simulink library "monroe_library"  (R2012b)
settings: Solver=ode45  StartTime=0.0  StopTime=10.0  RelTol=1e-3
values from neighbouring files (symbols this model uses):
  input_bit_width = ', num2str(input_bit_width))    [fft_direct_draw.m]
undefined symbols (not defined in the file or in its folder): gcbh, xlBlockLoadCallback
libraries: xbsIndex_r4 x1880, monroe_library x159, casper_library x13, xps_library x1
(part 42 of 43)

== system monroe_library/unscr_tail/mirror_spectrum/Subsystem3 ==
  In1 : Inport
  In3 : Inport  Port=2
  In4 : Inport  Port=3
  Delay11 : S-Function  LoadFcn=xlBlockLoadCallback(gcbh);  FunctionName=sysgen  Parameters=ptable_  EnableBusSupport=off  mask(Xilinx Delay Block){infoedit=Hardware notes: A delay line is a chain, each link of which is an SRL16 followed by a flip-flop., en_sgadvanced=, en=off, latency=1, dbl_ovrd_sgadvanced=, dbl_ovrd=off, reg_retiming_sgadvanced=, reg_retiming=off, xl_use_area_sgadvanced=, xl_use_area=off, xl_area=[0,0,0,0,0,0,0], has_advanced_control=0, sggui_pos=-1,-1,-1,-1, block_type=delay, block_version=, sg_icon_stat=25,28,1,1,white,blue,0,07b98262,right,,[ ],[ ], sg_mask_display=|, sg_list_contents=, sg_blockgui_xml=}
      mask sg_mask_display=|
      | fprintf('','COMMENT: begin icon graphics');
      | patch([0 25 25 0 0 ],[0 0 28 28 0 ],[0.77 0.82 0.91 ]);
      | plot([0 25 25 0 0 ],[0 0 28 28 0 ]);
      | patch([5.325 9.66 12.66 15.66 18.66 12.66 8.325 5.325 ],[17.33 17.33 20.33 17.33 20.33 20.33 20.33 17.33 ],[1 1 1 ]);
      | patch([8.325 12.66 9.66 5.325 8.325 ],[14.33 14.33 17.33 17.33 14.33 ],[0.931 0.946 0.973 ]);
      | patch([5.325 9.66 12.66 8.325 5.325 ],[11.33 11.33 14.33 14.33 11.33 ],[1 1 1 ]);
      | patch([8.325 18.66 15.66 12.66 9.66 5.325 8.325 ],[8.33 8.33 11.33 8.33 11.33 11.33 8.33 ],[0.931 0.946 0.973 ]);
      | fprintf('','COMMENT: end icon graphics');
      | fprintf('','COMMENT: begin icon text');
      |
      |
      | color('black');disp('z^{-1}','texmode','on');
      | fprintf('','COMMENT: end icon text');
      mask prompts: infoedit ""; en_sgadvanced ""; en "Provide enable port"; dbl_ovrd_sgadvanced ""; dbl_ovrd "Override with doubles"; reg_retiming_sgadvanced ""; reg_retiming "Implement using behavioral HDL."; xl_use_area_sgadvanced ""; xl_use_area "Define FPGA area for resource estimation"; xl_area "FPGA area [slices, FFs, BRAMs, LUTs, IOBs, emb. mults, TBUFs]"; has_advanced_control ""; sggui_pos ""; block_type ""; block_version ""; sg_icon_stat ""; sg_mask_display ""; sg_list_contents ""; sg_blockgui_xml ""
      mask help: Hardware notes: A delay line is a chain, each link of which is an SRL16 followed by a flip-flop.
      mask init: same as monroe_library/counter_limited_fast/Delay1
      settings: CopyFcn=xlBlockMoveCallback(gcbh);  DeleteFcn=xlDestroyGui(gcbh);  ModelCloseFcn=xlDestroyGui(gcbh);  PreSaveFcn=xlBlockPreSaveCallback(gcbh);  PostSaveFcn=xlBlockPostSaveCallback(gcbh);  DestroyFcn=xlDestroyGui(gcbh);  OpenFcn=xlOpenGui(gcbh, 'delay_gui.xml', @xlmagicenablement, -1)  CloseFcn=xlDestroyGui(gcbh);  MoveFcn=xlBlockMoveCallback(gcbh);
      mask Help: eval('');xlDoc('-book','sysgen','-topic','Delay');
      mask Display:
      | fprintf('','COMMENT: begin icon graphics');
      | patch([0 25 25 0 0 ],[0 0 28 28 0 ],[0.77 0.82 0.91 ]);
      | plot([0 25 25 0 0 ],[0 0 28 28 0 ]);
      | patch([5.325 9.66 12.66 15.66 18.66 12.66 8.325 5.325 ],[17.33 17.33 20.33 17.33 20.33 20.33 20.33 17.33 ],[1 1 1 ]);
      | patch([8.325 12.66 9.66 5.325 8.325 ],[14.33 14.33 17.33 17.33 14.33 ],[0.931 0.946 0.973 ]);
      | patch([5.325 9.66 12.66 8.325 5.325 ],[11.33 11.33 14.33 14.33 11.33 ],[1 1 1 ]);
      | patch([8.325 18.66 15.66 12.66 9.66 5.325 8.325 ],[8.33 8.33 11.33 8.33 11.33 11.33 8.33 ],[0.931 0.946 0.973 ]);
      | fprintf('','COMMENT: end icon graphics');
      | fprintf('','COMMENT: begin icon text');
      | 
      | 
      | color('black');disp('z^{-1}','texmode','on');
      | fprintf('','COMMENT: end icon text');
  Delay7 : xbsIndex_r4/Delay  en=off  latency=1  dbl_ovrd=off  reg_retiming=off  block_type=delay
  Mux4 : S-Function  LoadFcn=xlBlockLoadCallback(gcbh);  FunctionName=sysgen  Parameters=ptable_  EnableBusSupport=off  mask(Xilinx Bus Multiplexer Block){inputs_sgadvanced=, inputs=2, en_sgadvanced=, en=off, latency=0, precision_sgadvanced=, precision=Full, arith_type_sgadvanced=, arith_type=Signed  (2's comp), n_bits=8, bin_pt=2, quantization_sgadvanced=, quantization=Truncate, overflow_sgadvanced=, overflow=Wrap, dbl_ovrd_sgadvanced=, dbl_ovrd=off, xl_use_area_sgadvanced=, xl_use_area=off, xl_area=[0,0,0,0,0,0,0], infoedit=, has_advanced_control=0, sggui_pos=-1,-1,-1,-1, block_type=mux, block_version=, sg_icon_stat=45,104,3,1,white,blue,3,eb98d690,right,,[ ],[ ], sg_mask_display=|, sg_list_contents=, sg_blockgui_xml=}
      mask sg_mask_display=|
      | fprintf('','COMMENT: begin icon graphics');
      | patch([0 45 45 0 0 ],[0 14.8571 89.1429 104 0 ],[0.77 0.82 0.91 ]);
      | plot([0 45 45 0 0 ],[0 14.8571 89.1429 104 0 ]);
      | patch([8.65 17.32 23.32 29.32 35.32 23.32 14.65 8.65 ],[58.66 58.66 64.66 58.66 64.66 64.66 64.66 58.66 ],[1 1 1 ]);
      | patch([14.65 23.32 17.32 8.65 14.65 ],[52.66 52.66 58.66 58.66 52.66 ],[0.931 0.946 0.973 ]);
      | patch([8.65 17.32 23.32 14.65 8.65 ],[46.66 46.66 52.66 52.66 46.66 ],[1 1 1 ]);
      | patch([14.65 35.32 29.32 23.32 17.32 8.65 14.65 ],[40.66 40.66 46.66 40.66 46.66 46.66 40.66 ],[0.931 0.946 0.973 ]);
      | fprintf('','COMMENT: end icon graphics');
      | fprintf('','COMMENT: begin icon text');
      | color('black');port_label('input',1,'sel');
      | color('black');port_label('input',2,'d0');
      | color('black');port_label('input',3,'d1');
      |
      | color('black');disp('\bf{}','texmode','on');
      | fprintf('','COMMENT: end icon text');
      mask prompts: inputs_sgadvanced ""; inputs "Number of inputs"; en_sgadvanced ""; en "Provide enable port"; precision_sgadvanced ""; arith_type_sgadvanced ""; arith_type "Output type"; n_bits "Number of bits"; bin_pt "Binary point"; quantization_sgadvanced ""; overflow_sgadvanced ""; dbl_ovrd_sgadvanced ""; dbl_ovrd "Override with doubles"; xl_use_area_sgadvanced ""; xl_use_area "Define FPGA area for resource estimation"; xl_area "FPGA area [slices, FFs, BRAMs, LUTs, IOBs, emb. mults, TBUFs]"; infoedit ""; has_advanced_control ""; sggui_pos ""; block_type ""; block_version ""; sg_icon_stat ""; sg_mask_display ""; sg_list_contents ""; sg_blockgui_xml ""
      mask help: Xilinx Bus Multiplexer
      mask init: same as monroe_library/unscr_tail/mirror_spectrum/Subsystem/Mux4
      settings: CopyFcn=xlBlockMoveCallback(gcbh);  DeleteFcn=xlDestroyGui(gcbh);  ModelCloseFcn=xlDestroyGui(gcbh);  PreSaveFcn=xlBlockPreSaveCallback(gcbh);  PostSaveFcn=xlBlockPostSaveCallback(gcbh);  DestroyFcn=xlDestroyGui(gcbh);  OpenFcn=xlOpenGui(gcbh, 'mux_gui.xml', @muxenablement, -1)  CloseFcn=xlDestroyGui(gcbh);  MoveFcn=xlBlockMoveCallback(gcbh);
      mask Help: eval('');xlDoc('-book','sysgen','-topic','Mux');
      mask TypeOptions inputs: 2 | 3 | 4 | 5 | 6 | 7 | 8 | 9 | 10 | 11 | 12 | 13 | 14 | 15 | 16 | 17 | 18 | 19 | 20 | 21 | 22 | 23 | 24 | 25 | 26 | 27 | 28 | 29 | 30 | 31 | 32
      mask TypeOptions precision: Full | User Defined
      mask TypeOptions arith_type: Signed  (2's comp) | Unsigned
      mask TypeOptions quantization: Truncate | Round  (unbiased: +/- Inf)
      mask TypeOptions overflow: Wrap | Saturate | Flag as error
      mask Display:
      | fprintf('','COMMENT: begin icon graphics');
      | patch([0 45 45 0 0 ],[0 14.8571 89.1429 104 0 ],[0.77 0.82 0.91 ]);
      | plot([0 45 45 0 0 ],[0 14.8571 89.1429 104 0 ]);
      | patch([8.65 17.32 23.32 29.32 35.32 23.32 14.65 8.65 ],[58.66 58.66 64.66 58.66 64.66 64.66 64.66 58.66 ],[1 1 1 ]);
      | patch([14.65 23.32 17.32 8.65 14.65 ],[52.66 52.66 58.66 58.66 52.66 ],[0.931 0.946 0.973 ]);
      | patch([8.65 17.32 23.32 14.65 8.65 ],[46.66 46.66 52.66 52.66 46.66 ],[1 1 1 ]);
      | patch([14.65 35.32 29.32 23.32 17.32 8.65 14.65 ],[40.66 40.66 46.66 40.66 46.66 46.66 40.66 ],[0.931 0.946 0.973 ]);
      | fprintf('','COMMENT: end icon graphics');
      | fprintf('','COMMENT: begin icon text');
      | color('black');port_label('input',1,'sel');
      | color('black');port_label('input',2,'d0');
      | color('black');port_label('input',3,'d1');
      | 
      | color('black');disp('\bf{}','texmode','on');
      | fprintf('','COMMENT: end icon text');
  Mux5 : S-Function  LoadFcn=xlBlockLoadCallback(gcbh);  FunctionName=sysgen  Parameters=ptable_  EnableBusSupport=off  mask(Xilinx Bus Multiplexer Block){inputs_sgadvanced=, inputs=2, en_sgadvanced=, en=off, latency=0, precision_sgadvanced=, precision=Full, arith_type_sgadvanced=, arith_type=Signed  (2's comp), n_bits=8, bin_pt=2, quantization_sgadvanced=, quantization=Truncate, overflow_sgadvanced=, overflow=Wrap, dbl_ovrd_sgadvanced=, dbl_ovrd=off, xl_use_area_sgadvanced=, xl_use_area=off, xl_area=[0,0,0,0,0,0,0], infoedit=, has_advanced_control=0, sggui_pos=-1,-1,-1,-1, block_type=mux, block_version=, sg_icon_stat=45,104,3,1,white,blue,3,eb98d690,right,,[ ],[ ], sg_mask_display=|, sg_list_contents=, sg_blockgui_xml=}
      mask sg_mask_display=|
      | fprintf('','COMMENT: begin icon graphics');
      | patch([0 45 45 0 0 ],[0 14.8571 89.1429 104 0 ],[0.77 0.82 0.91 ]);
      | plot([0 45 45 0 0 ],[0 14.8571 89.1429 104 0 ]);
      | patch([8.65 17.32 23.32 29.32 35.32 23.32 14.65 8.65 ],[58.66 58.66 64.66 58.66 64.66 64.66 64.66 58.66 ],[1 1 1 ]);
      | patch([14.65 23.32 17.32 8.65 14.65 ],[52.66 52.66 58.66 58.66 52.66 ],[0.931 0.946 0.973 ]);
      | patch([8.65 17.32 23.32 14.65 8.65 ],[46.66 46.66 52.66 52.66 46.66 ],[1 1 1 ]);
      | patch([14.65 35.32 29.32 23.32 17.32 8.65 14.65 ],[40.66 40.66 46.66 40.66 46.66 46.66 40.66 ],[0.931 0.946 0.973 ]);
      | fprintf('','COMMENT: end icon graphics');
      | fprintf('','COMMENT: begin icon text');
      | color('black');port_label('input',1,'sel');
      | color('black');port_label('input',2,'d0');
      | color('black');port_label('input',3,'d1');
      |
      | color('black');disp('\bf{}','texmode','on');
      | fprintf('','COMMENT: end icon text');
      mask prompts: inputs_sgadvanced ""; inputs "Number of inputs"; en_sgadvanced ""; en "Provide enable port"; precision_sgadvanced ""; arith_type_sgadvanced ""; arith_type "Output type"; n_bits "Number of bits"; bin_pt "Binary point"; quantization_sgadvanced ""; overflow_sgadvanced ""; dbl_ovrd_sgadvanced ""; dbl_ovrd "Override with doubles"; xl_use_area_sgadvanced ""; xl_use_area "Define FPGA area for resource estimation"; xl_area "FPGA area [slices, FFs, BRAMs, LUTs, IOBs, emb. mults, TBUFs]"; infoedit ""; has_advanced_control ""; sggui_pos ""; block_type ""; block_version ""; sg_icon_stat ""; sg_mask_display ""; sg_list_contents ""; sg_blockgui_xml ""
      mask help: Xilinx Bus Multiplexer
      mask init: same as monroe_library/unscr_tail/mirror_spectrum/Subsystem/Mux4
      settings: CopyFcn=xlBlockMoveCallback(gcbh);  DeleteFcn=xlDestroyGui(gcbh);  ModelCloseFcn=xlDestroyGui(gcbh);  PreSaveFcn=xlBlockPreSaveCallback(gcbh);  PostSaveFcn=xlBlockPostSaveCallback(gcbh);  DestroyFcn=xlDestroyGui(gcbh);  OpenFcn=xlOpenGui(gcbh, 'mux_gui.xml', @muxenablement, -1)  CloseFcn=xlDestroyGui(gcbh);  MoveFcn=xlBlockMoveCallback(gcbh);
      mask Help: eval('');xlDoc('-book','sysgen','-topic','Mux');
      mask TypeOptions inputs: 2 | 3 | 4 | 5 | 6 | 7 | 8 | 9 | 10 | 11 | 12 | 13 | 14 | 15 | 16 | 17 | 18 | 19 | 20 | 21 | 22 | 23 | 24 | 25 | 26 | 27 | 28 | 29 | 30 | 31 | 32
      mask TypeOptions precision: Full | User Defined
      mask TypeOptions arith_type: Signed  (2's comp) | Unsigned
      mask TypeOptions quantization: Truncate | Round  (unbiased: +/- Inf)
      mask TypeOptions overflow: Wrap | Saturate | Flag as error
      mask Display:
      | fprintf('','COMMENT: begin icon graphics');
      | patch([0 45 45 0 0 ],[0 14.8571 89.1429 104 0 ],[0.77 0.82 0.91 ]);
      | plot([0 45 45 0 0 ],[0 14.8571 89.1429 104 0 ]);
      | patch([8.65 17.32 23.32 29.32 35.32 23.32 14.65 8.65 ],[58.66 58.66 64.66 58.66 64.66 64.66 64.66 58.66 ],[1 1 1 ]);
      | patch([14.65 23.32 17.32 8.65 14.65 ],[52.66 52.66 58.66 58.66 52.66 ],[0.931 0.946 0.973 ]);
      | patch([8.65 17.32 23.32 14.65 8.65 ],[46.66 46.66 52.66 52.66 46.66 ],[1 1 1 ]);
      | patch([14.65 35.32 29.32 23.32 17.32 8.65 14.65 ],[40.66 40.66 46.66 40.66 46.66 46.66 40.66 ],[0.931 0.946 0.973 ]);
      | fprintf('','COMMENT: end icon graphics');
      | fprintf('','COMMENT: begin icon text');
      | color('black');port_label('input',1,'sel');
      | color('black');port_label('input',2,'d0');
      | color('black');port_label('input',3,'d1');
      | 
      | color('black');disp('\bf{}','texmode','on');
      | fprintf('','COMMENT: end icon text');
  cram5 : Subsystem
  uncram5 : monroe_library/unscr_tail/mirror_spectrum/uncram1  SystemSampleTime=-1
  uncram6 : Subsystem
  Out1 : Outport
  wires:
  In4/1 -> uncram6/1(in)
  In3/1 -> uncram5/1
  cram5/1(out) -> Out1/1
  In1/1 -> Delay7/1, Delay11/1
  Mux4/1 -> cram5/1(in0)
  Mux5/1 -> cram5/2(in1)
  Delay7/1 -> Mux5/1
  Delay11/1 -> Mux4/1
  uncram6/2(out1) -> Mux5/3
  uncram5/2 -> Mux5/2
  uncram6/1(out0) -> Mux4/3
  uncram5/1 -> Mux4/2

== system monroe_library/unscr_tail/mirror_spectrum/cram1 ==
  in0 : Inport
  in1 : Inport  Port=2
  Concat5 : xbsIndex_r4/Concat  num_inputs=2  dbl_ovrd=off  block_type=concat
  Reinterpret23 : xbsIndex_r4/Reinterpret  force_arith_type=on  arith_type=Unsigned  force_bin_pt=on  bin_pt=0  block_type=reinterpret
      settings: infoedit="Changes signal type without altering the binary representation.   You can changed the signal between signed and unsigned, and relocate the binary point.<br><br>Hardware notes: In hardware this block costs nothing.<br><br>Example:  Suppose the input is 6 bits wide, signed, with 2 fractional bits, and the output is forced to unsigned with 0 fractional bits.  Then an input of -2.0 (1110.00 in binary 2's complement) becomes an output of 56 (111000 in binary)."
  Reinterpret24 : xbsIndex_r4/Reinterpret  force_arith_type=on  arith_type=Unsigned  force_bin_pt=on  bin_pt=0  block_type=reinterpret
      settings: infoedit="Changes signal type without altering the binary representation.   You can changed the signal between signed and unsigned, and relocate the binary point.<br><br>Hardware notes: In hardware this block costs nothing.<br><br>Example:  Suppose the input is 6 bits wide, signed, with 2 fractional bits, and the output is forced to unsigned with 0 fractional bits.  Then an input of -2.0 (1110.00 in binary 2's complement) becomes an output of 56 (111000 in binary)."
  out : Outport
  wires:
  Reinterpret24/1 -> Concat5/2
  in1/1 -> Reinterpret24/1
  Reinterpret23/1 -> Concat5/1
  in0/1 -> Reinterpret23/1
  Concat5/1 -> out/1

== system monroe_library/unscr_tail/mirror_spectrum/cram2 ==
  in0 : Inport
  in1 : Inport  Port=2
  Concat6 : xbsIndex_r4/Concat  num_inputs=2  dbl_ovrd=off  block_type=concat
  Reinterpret25 : xbsIndex_r4/Reinterpret  force_arith_type=on  arith_type=Unsigned  force_bin_pt=on  bin_pt=0  block_type=reinterpret
      settings: infoedit="Changes signal type without altering the binary representation.   You can changed the signal between signed and unsigned, and relocate the binary point.<br><br>Hardware notes: In hardware this block costs nothing.<br><br>Example:  Suppose the input is 6 bits wide, signed, with 2 fractional bits, and the output is forced to unsigned with 0 fractional bits.  Then an input of -2.0 (1110.00 in binary 2's complement) becomes an output of 56 (111000 in binary)."
  Reinterpret26 : xbsIndex_r4/Reinterpret  force_arith_type=on  arith_type=Unsigned  force_bin_pt=on  bin_pt=0  block_type=reinterpret
      settings: infoedit="Changes signal type without altering the binary representation.   You can changed the signal between signed and unsigned, and relocate the binary point.<br><br>Hardware notes: In hardware this block costs nothing.<br><br>Example:  Suppose the input is 6 bits wide, signed, with 2 fractional bits, and the output is forced to unsigned with 0 fractional bits.  Then an input of -2.0 (1110.00 in binary 2's complement) becomes an output of 56 (111000 in binary)."
  out : Outport
  wires:
  Reinterpret26/1 -> Concat6/2
  in1/1 -> Reinterpret26/1
  Reinterpret25/1 -> Concat6/1
  in0/1 -> Reinterpret25/1
  Concat6/1 -> out/1

== system monroe_library/unscr_tail/mirror_spectrum/cram3 ==
  in0 : Inport
  in1 : Inport  Port=2
  Concat7 : xbsIndex_r4/Concat  num_inputs=2  dbl_ovrd=off  block_type=concat
  Reinterpret27 : xbsIndex_r4/Reinterpret  force_arith_type=on  arith_type=Unsigned  force_bin_pt=on  bin_pt=0  block_type=reinterpret
      settings: infoedit="Changes signal type without altering the binary representation.   You can changed the signal between signed and unsigned, and relocate the binary point.<br><br>Hardware notes: In hardware this block costs nothing.<br><br>Example:  Suppose the input is 6 bits wide, signed, with 2 fractional bits, and the output is forced to unsigned with 0 fractional bits.  Then an input of -2.0 (1110.00 in binary 2's complement) becomes an output of 56 (111000 in binary)."
  Reinterpret28 : xbsIndex_r4/Reinterpret  force_arith_type=on  arith_type=Unsigned  force_bin_pt=on  bin_pt=0  block_type=reinterpret
      settings: infoedit="Changes signal type without altering the binary representation.   You can changed the signal between signed and unsigned, and relocate the binary point.<br><br>Hardware notes: In hardware this block costs nothing.<br><br>Example:  Suppose the input is 6 bits wide, signed, with 2 fractional bits, and the output is forced to unsigned with 0 fractional bits.  Then an input of -2.0 (1110.00 in binary 2's complement) becomes an output of 56 (111000 in binary)."
  out : Outport
  wires:
  Reinterpret28/1 -> Concat7/2
  in1/1 -> Reinterpret28/1
  Reinterpret27/1 -> Concat7/1
  in0/1 -> Reinterpret27/1
  Concat7/1 -> out/1

== system monroe_library/unscr_tail/mirror_spectrum/cram4 ==
  in0 : Inport
  in1 : Inport  Port=2
  Concat8 : xbsIndex_r4/Concat  num_inputs=2  dbl_ovrd=off  block_type=concat
  Reinterpret29 : xbsIndex_r4/Reinterpret  force_arith_type=on  arith_type=Unsigned  force_bin_pt=on  bin_pt=0  block_type=reinterpret
      settings: infoedit="Changes signal type without altering the binary representation.   You can changed the signal between signed and unsigned, and relocate the binary point.<br><br>Hardware notes: In hardware this block costs nothing.<br><br>Example:  Suppose the input is 6 bits wide, signed, with 2 fractional bits, and the output is forced to unsigned with 0 fractional bits.  Then an input of -2.0 (1110.00 in binary 2's complement) becomes an output of 56 (111000 in binary)."
  Reinterpret30 : xbsIndex_r4/Reinterpret  force_arith_type=on  arith_type=Unsigned  force_bin_pt=on  bin_pt=0  block_type=reinterpret
      settings: infoedit="Changes signal type without altering the binary representation.   You can changed the signal between signed and unsigned, and relocate the binary point.<br><br>Hardware notes: In hardware this block costs nothing.<br><br>Example:  Suppose the input is 6 bits wide, signed, with 2 fractional bits, and the output is forced to unsigned with 0 fractional bits.  Then an input of -2.0 (1110.00 in binary 2's complement) becomes an output of 56 (111000 in binary)."
  out : Outport
  wires:
  Reinterpret30/1 -> Concat8/2
  in1/1 -> Reinterpret30/1
  Reinterpret29/1 -> Concat8/1
  in0/1 -> Reinterpret29/1
  Concat8/1 -> out/1

== system monroe_library/unscr_tail/mirror_spectrum/sel_gen ==
  sync_in : Inport
  Constant3 : xbsIndex_r4/Constant  arith_type=Unsigned  const=2^(FFTSize-1)  n_bits=FFTSize  bin_pt=0  explicit_period=on  period=1  equ=P=C  opselect=C  inp2=PCIN>>17  opr=+  inp1=P  carry=CIN  dbl_ovrd=off  block_type=constant
  Counter : xbsIndex_r4/Counter  cnt_type=Free Running  cnt_to=Inf  operation=Up  start_count=(2^FFTSize)-1  cnt_by_val=1  arith_type=Unsigned  n_bits=FFTSize  bin_pt=0  load_pin=off  rst=on  en=off  explicit_period=off  period=1  dbl_ovrd=off  use_behavioral_HDL=off  implementation=Fabric  use_rpm=on  block_type=counter
  Relational : xbsIndex_r4/Relational  mode=a>b  en=off  latency=1  dbl_ovrd=off  block_type=relational
  sel_out : Outport
  wires:
  Relational/1 -> sel_out/1
  Constant3/1 -> Relational/2
  Counter/1 -> Relational/1
  sync_in/1 -> Counter/1

== system monroe_library/unscr_tail/mirror_spectrum/uncram1 ==
  in : Inport
  Reinterpret15 : xbsIndex_r4/Reinterpret  force_arith_type=on  arith_type="Signed  (2's comp)"  force_bin_pt=on  bin_pt=input_bit_width-1  block_type=reinterpret
      settings: infoedit="Changes signal type without altering the binary representation.   You can changed the signal between signed and unsigned, and relocate the binary point.<br><br>Hardware notes: In hardware this block costs nothing.<br><br>Example:  Suppose the input is 6 bits wide, signed, with 2 fractional bits, and the output is forced to unsigned with 0 fractional bits.  Then an input of -2.0 (1110.00 in binary 2's complement) becomes an output of 56 (111000 in binary)."
  Reinterpret16 : xbsIndex_r4/Reinterpret  force_arith_type=on  arith_type="Signed  (2's comp)"  force_bin_pt=on  bin_pt=input_bit_width-1  block_type=reinterpret
      settings: infoedit="Changes signal type without altering the binary representation.   You can changed the signal between signed and unsigned, and relocate the binary point.<br><br>Hardware notes: In hardware this block costs nothing.<br><br>Example:  Suppose the input is 6 bits wide, signed, with 2 fractional bits, and the output is forced to unsigned with 0 fractional bits.  Then an input of -2.0 (1110.00 in binary 2's complement) becomes an output of 56 (111000 in binary)."
  Slice16 : xbsIndex_r4/Slice  nbits=input_bit_width  boolean_output=off  mode=Upper Bit Location + Width  bit1=-0  base1=MSB of Input  bit0=0  base0=MSB of Input  dbl_ovrd=off  block_type=slice
  Slice17 : xbsIndex_r4/Slice  nbits=input_bit_width  boolean_output=off  mode=Upper Bit Location + Width  bit1=-1* input_bit_width  base1=MSB of Input  bit0=0  base0=MSB of Input  dbl_ovrd=off  block_type=slice
  out0 : Outport
  out1 : Outport  Port=2
  wires:
  in/1 -> Slice17/1, Slice16/1
  Reinterpret16/1 -> out1/1
  Slice17/1 -> Reinterpret16/1
  Reinterpret15/1 -> out0/1
  Slice16/1 -> Reinterpret15/1

== system monroe_library/unscr_tail/mirror_spectrum/uncram2 ==
  in : Inport
  Reinterpret15 : xbsIndex_r4/Reinterpret  force_arith_type=on  arith_type="Signed  (2's comp)"  force_bin_pt=on  bin_pt=input_bit_width-1  block_type=reinterpret
      settings: infoedit="Changes signal type without altering the binary representation.   You can changed the signal between signed and unsigned, and relocate the binary point.<br><br>Hardware notes: In hardware this block costs nothing.<br><br>Example:  Suppose the input is 6 bits wide, signed, with 2 fractional bits, and the output is forced to unsigned with 0 fractional bits.  Then an input of -2.0 (1110.00 in binary 2's complement) becomes an output of 56 (111000 in binary)."
  Reinterpret16 : xbsIndex_r4/Reinterpret  force_arith_type=on  arith_type="Signed  (2's comp)"  force_bin_pt=on  bin_pt=input_bit_width-1  block_type=reinterpret
      settings: infoedit="Changes signal type without altering the binary representation.   You can changed the signal between signed and unsigned, and relocate the binary point.<br><br>Hardware notes: In hardware this block costs nothing.<br><br>Example:  Suppose the input is 6 bits wide, signed, with 2 fractional bits, and the output is forced to unsigned with 0 fractional bits.  Then an input of -2.0 (1110.00 in binary 2's complement) becomes an output of 56 (111000 in binary)."
  Slice16 : xbsIndex_r4/Slice  nbits=input_bit_width  boolean_output=off  mode=Upper Bit Location + Width  bit1=-0  base1=MSB of Input  bit0=0  base0=MSB of Input  dbl_ovrd=off  block_type=slice
  Slice17 : xbsIndex_r4/Slice  nbits=input_bit_width  boolean_output=off  mode=Upper Bit Location + Width  bit1=-1* input_bit_width  base1=MSB of Input  bit0=0  base0=MSB of Input  dbl_ovrd=off  block_type=slice
  out0 : Outport
  out1 : Outport  Port=2
  wires:
  Slice16/1 -> Reinterpret15/1
  Reinterpret15/1 -> out0/1
  Slice17/1 -> Reinterpret16/1
  Reinterpret16/1 -> out1/1
  in/1 -> Slice16/1, Slice17/1

== system monroe_library/unscr_tail/mirror_spectrum/uncram3 ==
  in : Inport
  Reinterpret15 : xbsIndex_r4/Reinterpret  force_arith_type=on  arith_type="Signed  (2's comp)"  force_bin_pt=on  bin_pt=input_bit_width-1  block_type=reinterpret
      settings: infoedit="Changes signal type without altering the binary representation.   You can changed the signal between signed and unsigned, and relocate the binary point.<br><br>Hardware notes: In hardware this block costs nothing.<br><br>Example:  Suppose the input is 6 bits wide, signed, with 2 fractional bits, and the output is forced to unsigned with 0 fractional bits.  Then an input of -2.0 (1110.00 in binary 2's complement) becomes an output of 56 (111000 in binary)."
  Reinterpret16 : xbsIndex_r4/Reinterpret  force_arith_type=on  arith_type="Signed  (2's comp)"  force_bin_pt=on  bin_pt=input_bit_width-1  block_type=reinterpret
      settings: infoedit="Changes signal type without altering the binary representation.   You can changed the signal between signed and unsigned, and relocate the binary point.<br><br>Hardware notes: In hardware this block costs nothing.<br><br>Example:  Suppose the input is 6 bits wide, signed, with 2 fractional bits, and the output is forced to unsigned with 0 fractional bits.  Then an input of -2.0 (1110.00 in binary 2's complement) becomes an output of 56 (111000 in binary)."
  Slice16 : xbsIndex_r4/Slice  nbits=input_bit_width  boolean_output=off  mode=Upper Bit Location + Width  bit1=-0  base1=MSB of Input  bit0=0  base0=MSB of Input  dbl_ovrd=off  block_type=slice
  Slice17 : xbsIndex_r4/Slice  nbits=input_bit_width  boolean_output=off  mode=Upper Bit Location + Width  bit1=-1* input_bit_width  base1=MSB of Input  bit0=0  base0=MSB of Input  dbl_ovrd=off  block_type=slice
  out0 : Outport
  out1 : Outport  Port=2
  wires:
  in/1 -> Slice17/1, Slice16/1
  Reinterpret16/1 -> out1/1
  Slice17/1 -> Reinterpret16/1
  Reinterpret15/1 -> out0/1
  Slice16/1 -> Reinterpret15/1

== system monroe_library/unscr_tail/mirror_spectrum/uncram4 ==
  in : Inport
  Reinterpret15 : xbsIndex_r4/Reinterpret  force_arith_type=on  arith_type="Signed  (2's comp)"  force_bin_pt=on  bin_pt=input_bit_width-1  block_type=reinterpret
      settings: infoedit="Changes signal type without altering the binary representation.   You can changed the signal between signed and unsigned, and relocate the binary point.<br><br>Hardware notes: In hardware this block costs nothing.<br><br>Example:  Suppose the input is 6 bits wide, signed, with 2 fractional bits, and the output is forced to unsigned with 0 fractional bits.  Then an input of -2.0 (1110.00 in binary 2's complement) becomes an output of 56 (111000 in binary)."
  Reinterpret16 : xbsIndex_r4/Reinterpret  force_arith_type=on  arith_type="Signed  (2's comp)"  force_bin_pt=on  bin_pt=input_bit_width-1  block_type=reinterpret
      settings: infoedit="Changes signal type without altering the binary representation.   You can changed the signal between signed and unsigned, and relocate the binary point.<br><br>Hardware notes: In hardware this block costs nothing.<br><br>Example:  Suppose the input is 6 bits wide, signed, with 2 fractional bits, and the output is forced to unsigned with 0 fractional bits.  Then an input of -2.0 (1110.00 in binary 2's complement) becomes an output of 56 (111000 in binary)."
  Slice16 : xbsIndex_r4/Slice  nbits=input_bit_width  boolean_output=off  mode=Upper Bit Location + Width  bit1=-0  base1=MSB of Input  bit0=0  base0=MSB of Input  dbl_ovrd=off  block_type=slice
  Slice17 : xbsIndex_r4/Slice  nbits=input_bit_width  boolean_output=off  mode=Upper Bit Location + Width  bit1=-1* input_bit_width  base1=MSB of Input  bit0=0  base0=MSB of Input  dbl_ovrd=off  block_type=slice
  out0 : Outport
  out1 : Outport  Port=2
  wires:
  Slice16/1 -> Reinterpret15/1
  Reinterpret15/1 -> out0/1
  Slice17/1 -> Reinterpret16/1
  Reinterpret16/1 -> out1/1
  in/1 -> Slice16/1, Slice17/1

== system monroe_library/unscr_tail/reorder2/addresser ==
  sync_in : Inport
  Counter : xbsIndex_r4/Counter  cnt_type=Free Running  cnt_to=1023  operation=Up  start_count=0  cnt_by_val=1  arith_type=Unsigned  n_bits=FFTSize  bin_pt=0  load_pin=off  rst=on  en=off  explicit_period=off  period=1  dbl_ovrd=off  use_behavioral_HDL=off  implementation=Fabric  use_rpm=on  block_type=counter
  Counter1 : xbsIndex_r4/Counter  cnt_type=Free Running  cnt_to=1023  operation=Down  start_count=(2^(FFTSize-1)) -1  cnt_by_val=1  arith_type=Unsigned  n_bits=FFTSize-1  bin_pt=0  load_pin=off  rst=on  en=off  explicit_period=off  period=1  dbl_ovrd=off  use_behavioral_HDL=off  implementation=Fabric  use_rpm=on  block_type=counter
  Mux : xbsIndex_r4/Mux  inputs=2  en=off  latency=0  precision=Full  arith_type="Signed  (2's comp)"  n_bits=8  bin_pt=2  quantization=Truncate  overflow=Wrap  dbl_ovrd=off  block_type=mux
  Slice1 : xbsIndex_r4/Slice  nbits=1  boolean_output=off  mode=Upper Bit Location + Width  bit1=0  base1=MSB of Input  bit0=0  base0=LSB of Input  dbl_ovrd=off  block_type=slice
  Slice2 : xbsIndex_r4/Slice  nbits=FFTSize-1  boolean_output=off  mode=Lower Bit Location + Width  bit1=0  base1=MSB of Input  bit0=0  base0=LSB of Input  dbl_ovrd=off  block_type=slice
  addr_out : Outport
  wires:
  sync_in/1 -> Counter1/1, Counter/1
  Counter/1 -> Slice2/1, Slice1/1
  Slice2/1 -> Mux/2
  Slice1/1 -> Mux/1
  Mux/1 -> addr_out/1
  Counter1/1 -> Mux/3

== system monroe_library/unscr_tail/reorder2/addresser1 ==
  sync_in : Inport
  Counter : xbsIndex_r4/Counter  cnt_type=Free Running  cnt_to=1023  operation=Up  start_count=0  cnt_by_val=1  arith_type=Unsigned  n_bits=FFTSize  bin_pt=0  load_pin=off  rst=on  en=off  explicit_period=off  period=1  dbl_ovrd=off  use_behavioral_HDL=off  implementation=Fabric  use_rpm=on  block_type=counter
  Counter1 : xbsIndex_r4/Counter  cnt_type=Free Running  cnt_to=1023  operation=Down  start_count=(2^(FFTSize-1)) -1  cnt_by_val=1  arith_type=Unsigned  n_bits=FFTSize-1  bin_pt=0  load_pin=off  rst=on  en=off  explicit_period=off  period=1  dbl_ovrd=off  use_behavioral_HDL=off  implementation=Fabric  use_rpm=on  block_type=counter
  Mux : xbsIndex_r4/Mux  inputs=2  en=off  latency=0  precision=Full  arith_type="Signed  (2's comp)"  n_bits=8  bin_pt=2  quantization=Truncate  overflow=Wrap  dbl_ovrd=off  block_type=mux
  Slice1 : xbsIndex_r4/Slice  nbits=1  boolean_output=off  mode=Upper Bit Location + Width  bit1=0  base1=MSB of Input  bit0=0  base0=LSB of Input  dbl_ovrd=off  block_type=slice
  Slice2 : xbsIndex_r4/Slice  nbits=FFTSize-1  boolean_output=off  mode=Lower Bit Location + Width  bit1=0  base1=MSB of Input  bit0=0  base0=LSB of Input  dbl_ovrd=off  block_type=slice
  addr_out : Outport
  wires:
  Counter1/1 -> Mux/3
  Mux/1 -> addr_out/1
  Slice1/1 -> Mux/1
  Slice2/1 -> Mux/2
  Counter/1 -> Slice1/1, Slice2/1
  sync_in/1 -> Counter/1, Counter1/1

== system monroe_library/unscr_tail/reorder2/sync_tree ==
  In1 : Inport
  Delay{7..13} (7 alike) : xbsIndex_r4/Delay  en=off  latency=1  dbl_ovrd=off  reg_retiming=off  block_type=delay
  Out1 : Outport
  Out2 : Outport  Port=2
  Out3 : Outport  Port=3
  Out4 : Outport  Port=4
  wires:
  Delay7/1 -> Delay9/1, Delay8/1
  Delay8/1 -> Delay13/1, Delay12/1
  Delay9/1 -> Delay11/1, Delay10/1
  In1/1 -> Delay7/1
  Delay13/1 -> Out1/1
  Delay12/1 -> Out2/1
  Delay11/1 -> Out3/1
  Delay10/1 -> Out4/1

== system monroe_library/FFT_Biplex_4x/biplex_4x_unscr/dual_bit_reverse/bit_reverse_1 ==
  in : Inport
  concat : xbsIndex_r4/Concat  num_inputs=9  dbl_ovrd=off  block_type=concat
  slice1 : xbsIndex_r4/Slice  nbits=1  boolean_output=on  mode=Upper Bit Location + Width  bit1=-0  base1=MSB of Input  bit0=-0  base0=MSB of Input  dbl_ovrd=off  block_type=slice
  slice2 : xbsIndex_r4/Slice  nbits=1  boolean_output=on  mode=Upper Bit Location + Width  bit1=-1  base1=MSB of Input  bit0=-1  base0=MSB of Input  dbl_ovrd=off  block_type=slice
  slice3 : xbsIndex_r4/Slice  nbits=1  boolean_output=on  mode=Upper Bit Location + Width  bit1=-2  base1=MSB of Input  bit0=-2  base0=MSB of Input  dbl_ovrd=off  block_type=slice
  slice4 : xbsIndex_r4/Slice  nbits=1  boolean_output=on  mode=Upper Bit Location + Width  bit1=-3  base1=MSB of Input  bit0=-3  base0=MSB of Input  dbl_ovrd=off  block_type=slice
  slice5 : xbsIndex_r4/Slice  nbits=1  boolean_output=on  mode=Upper Bit Location + Width  bit1=-4  base1=MSB of Input  bit0=-4  base0=MSB of Input  dbl_ovrd=off  block_type=slice
  slice6 : xbsIndex_r4/Slice  nbits=1  boolean_output=on  mode=Upper Bit Location + Width  bit1=-5  base1=MSB of Input  bit0=-5  base0=MSB of Input  dbl_ovrd=off  block_type=slice
  slice7 : xbsIndex_r4/Slice  nbits=1  boolean_output=on  mode=Upper Bit Location + Width  bit1=-6  base1=MSB of Input  bit0=-6  base0=MSB of Input  dbl_ovrd=off  block_type=slice
  slice8 : xbsIndex_r4/Slice  nbits=1  boolean_output=on  mode=Upper Bit Location + Width  bit1=-7  base1=MSB of Input  bit0=-7  base0=MSB of Input  dbl_ovrd=off  block_type=slice
  slice9 : xbsIndex_r4/Slice  nbits=1  boolean_output=on  mode=Upper Bit Location + Width  bit1=-8  base1=MSB of Input  bit0=-8  base0=MSB of Input  dbl_ovrd=off  block_type=slice
  out : Outport
  wires:
  in/1 -> slice9/1, slice8/1, slice7/1, slice6/1, slice5/1, slice4/1, slice3/1, slice2/1, slice1/1
  concat/1 -> out/1
  slice1/1 -> concat/9
  slice2/1 -> concat/8
  slice3/1 -> concat/7
  slice4/1 -> concat/6
  slice5/1 -> concat/5
  slice6/1 -> concat/4
  slice7/1 -> concat/3
  slice8/1 -> concat/2
  slice9/1 -> concat/1

== system monroe_library/FFT_Biplex_4x/biplex_4x_unscr/dual_bit_reverse/bit_reverse_2 ==
  in : Inport
  concat : xbsIndex_r4/Concat  num_inputs=9  dbl_ovrd=off  block_type=concat
  slice1 : xbsIndex_r4/Slice  nbits=1  boolean_output=on  mode=Upper Bit Location + Width  bit1=-0  base1=MSB of Input  bit0=-0  base0=MSB of Input  dbl_ovrd=off  block_type=slice
  slice2 : xbsIndex_r4/Slice  nbits=1  boolean_output=on  mode=Upper Bit Location + Width  bit1=-1  base1=MSB of Input  bit0=-1  base0=MSB of Input  dbl_ovrd=off  block_type=slice
  slice3 : xbsIndex_r4/Slice  nbits=1  boolean_output=on  mode=Upper Bit Location + Width  bit1=-2  base1=MSB of Input  bit0=-2  base0=MSB of Input  dbl_ovrd=off  block_type=slice
  slice4 : xbsIndex_r4/Slice  nbits=1  boolean_output=on  mode=Upper Bit Location + Width  bit1=-3  base1=MSB of Input  bit0=-3  base0=MSB of Input  dbl_ovrd=off  block_type=slice
  slice5 : xbsIndex_r4/Slice  nbits=1  boolean_output=on  mode=Upper Bit Location + Width  bit1=-4  base1=MSB of Input  bit0=-4  base0=MSB of Input  dbl_ovrd=off  block_type=slice
  slice6 : xbsIndex_r4/Slice  nbits=1  boolean_output=on  mode=Upper Bit Location + Width  bit1=-5  base1=MSB of Input  bit0=-5  base0=MSB of Input  dbl_ovrd=off  block_type=slice
  slice7 : xbsIndex_r4/Slice  nbits=1  boolean_output=on  mode=Upper Bit Location + Width  bit1=-6  base1=MSB of Input  bit0=-6  base0=MSB of Input  dbl_ovrd=off  block_type=slice
  slice8 : xbsIndex_r4/Slice  nbits=1  boolean_output=on  mode=Upper Bit Location + Width  bit1=-7  base1=MSB of Input  bit0=-7  base0=MSB of Input  dbl_ovrd=off  block_type=slice
  slice9 : xbsIndex_r4/Slice  nbits=1  boolean_output=on  mode=Upper Bit Location + Width  bit1=-8  base1=MSB of Input  bit0=-8  base0=MSB of Input  dbl_ovrd=off  block_type=slice
  out : Outport
  wires:
  in/1 -> slice9/1, slice8/1, slice7/1, slice6/1, slice5/1, slice4/1, slice3/1, slice2/1, slice1/1
  concat/1 -> out/1
  slice1/1 -> concat/9
  slice2/1 -> concat/8
  slice3/1 -> concat/7
  slice4/1 -> concat/6
  slice5/1 -> concat/5
  slice6/1 -> concat/4
  slice7/1 -> concat/3
  slice8/1 -> concat/2
  slice9/1 -> concat/1

== system monroe_library/unscr_tail/mirror_spectrum/Subsystem/cram5 ==
  in0 : Inport
  in1 : Inport  Port=2
  Concat5 : xbsIndex_r4/Concat  num_inputs=2  dbl_ovrd=off  block_type=concat
  Reinterpret23 : xbsIndex_r4/Reinterpret  force_arith_type=on  arith_type=Unsigned  force_bin_pt=on  bin_pt=0  block_type=reinterpret
      settings: infoedit="Changes signal type without altering the binary representation.   You can changed the signal between signed and unsigned, and relocate the binary point.<br><br>Hardware notes: In hardware this block costs nothing.<br><br>Example:  Suppose the input is 6 bits wide, signed, with 2 fractional bits, and the output is forced to unsigned with 0 fractional bits.  Then an input of -2.0 (1110.00 in binary 2's complement) becomes an output of 56 (111000 in binary)."
  Reinterpret24 : xbsIndex_r4/Reinterpret  force_arith_type=on  arith_type=Unsigned  force_bin_pt=on  bin_pt=0  block_type=reinterpret
      settings: infoedit="Changes signal type without altering the binary representation.   You can changed the signal between signed and unsigned, and relocate the binary point.<br><br>Hardware notes: In hardware this block costs nothing.<br><br>Example:  Suppose the input is 6 bits wide, signed, with 2 fractional bits, and the output is forced to unsigned with 0 fractional bits.  Then an input of -2.0 (1110.00 in binary 2's complement) becomes an output of 56 (111000 in binary)."
  out : Outport
  wires:
  Concat5/1 -> out/1
  in0/1 -> Reinterpret23/1
  Reinterpret23/1 -> Concat5/1
  in1/1 -> Reinterpret24/1
  Reinterpret24/1 -> Concat5/2

== system monroe_library/unscr_tail/mirror_spectrum/Subsystem/uncram6 ==
  in : Inport
  Reinterpret15 : xbsIndex_r4/Reinterpret  force_arith_type=on  arith_type="Signed  (2's comp)"  force_bin_pt=on  bin_pt=input_bit_width-1  block_type=reinterpret
      settings: infoedit="Changes signal type without altering the binary representation.   You can changed the signal between signed and unsigned, and relocate the binary point.<br><br>Hardware notes: In hardware this block costs nothing.<br><br>Example:  Suppose the input is 6 bits wide, signed, with 2 fractional bits, and the output is forced to unsigned with 0 fractional bits.  Then an input of -2.0 (1110.00 in binary 2's complement) becomes an output of 56 (111000 in binary)."
  Reinterpret16 : xbsIndex_r4/Reinterpret  force_arith_type=on  arith_type="Signed  (2's comp)"  force_bin_pt=on  bin_pt=input_bit_width-1  block_type=reinterpret
      settings: infoedit="Changes signal type without altering the binary representation.   You can changed the signal between signed and unsigned, and relocate the binary point.<br><br>Hardware notes: In hardware this block costs nothing.<br><br>Example:  Suppose the input is 6 bits wide, signed, with 2 fractional bits, and the output is forced to unsigned with 0 fractional bits.  Then an input of -2.0 (1110.00 in binary 2's complement) becomes an output of 56 (111000 in binary)."
  Slice16 : xbsIndex_r4/Slice  nbits=input_bit_width  boolean_output=off  mode=Upper Bit Location + Width  bit1=-0  base1=MSB of Input  bit0=0  base0=MSB of Input  dbl_ovrd=off  block_type=slice
  Slice17 : xbsIndex_r4/Slice  nbits=input_bit_width  boolean_output=off  mode=Upper Bit Location + Width  bit1=-1* input_bit_width  base1=MSB of Input  bit0=0  base0=MSB of Input  dbl_ovrd=off  block_type=slice
  out0 : Outport
  out1 : Outport  Port=2
  wires:
  Slice16/1 -> Reinterpret15/1
  Reinterpret15/1 -> out0/1
  Slice17/1 -> Reinterpret16/1
  Reinterpret16/1 -> out1/1
  in/1 -> Slice16/1, Slice17/1

== system monroe_library/unscr_tail/mirror_spectrum/Subsystem1/cram5 ==
  in0 : Inport
  in1 : Inport  Port=2
  Concat5 : xbsIndex_r4/Concat  num_inputs=2  dbl_ovrd=off  block_type=concat
  Reinterpret23 : xbsIndex_r4/Reinterpret  force_arith_type=on  arith_type=Unsigned  force_bin_pt=on  bin_pt=0  block_type=reinterpret
      settings: infoedit="Changes signal type without altering the binary representation.   You can changed the signal between signed and unsigned, and relocate the binary point.<br><br>Hardware notes: In hardware this block costs nothing.<br><br>Example:  Suppose the input is 6 bits wide, signed, with 2 fractional bits, and the output is forced to unsigned with 0 fractional bits.  Then an input of -2.0 (1110.00 in binary 2's complement) becomes an output of 56 (111000 in binary)."
  Reinterpret24 : xbsIndex_r4/Reinterpret  force_arith_type=on  arith_type=Unsigned  force_bin_pt=on  bin_pt=0  block_type=reinterpret
      settings: infoedit="Changes signal type without altering the binary representation.   You can changed the signal between signed and unsigned, and relocate the binary point.<br><br>Hardware notes: In hardware this block costs nothing.<br><br>Example:  Suppose the input is 6 bits wide, signed, with 2 fractional bits, and the output is forced to unsigned with 0 fractional bits.  Then an input of -2.0 (1110.00 in binary 2's complement) becomes an output of 56 (111000 in binary)."
  out : Outport
  wires:
  Reinterpret24/1 -> Concat5/2
  in1/1 -> Reinterpret24/1
  Reinterpret23/1 -> Concat5/1
  in0/1 -> Reinterpret23/1
  Concat5/1 -> out/1

== system monroe_library/unscr_tail/mirror_spectrum/Subsystem1/uncram6 ==
  in : Inport
  Reinterpret15 : xbsIndex_r4/Reinterpret  force_arith_type=on  arith_type="Signed  (2's comp)"  force_bin_pt=on  bin_pt=input_bit_width-1  block_type=reinterpret
      settings: infoedit="Changes signal type without altering the binary representation.   You can changed the signal between signed and unsigned, and relocate the binary point.<br><br>Hardware notes: In hardware this block costs nothing.<br><br>Example:  Suppose the input is 6 bits wide, signed, with 2 fractional bits, and the output is forced to unsigned with 0 fractional bits.  Then an input of -2.0 (1110.00 in binary 2's complement) becomes an output of 56 (111000 in binary)."
  Reinterpret16 : xbsIndex_r4/Reinterpret  force_arith_type=on  arith_type="Signed  (2's comp)"  force_bin_pt=on  bin_pt=input_bit_width-1  block_type=reinterpret
      settings: infoedit="Changes signal type without altering the binary representation.   You can changed the signal between signed and unsigned, and relocate the binary point.<br><br>Hardware notes: In hardware this block costs nothing.<br><br>Example:  Suppose the input is 6 bits wide, signed, with 2 fractional bits, and the output is forced to unsigned with 0 fractional bits.  Then an input of -2.0 (1110.00 in binary 2's complement) becomes an output of 56 (111000 in binary)."
  Slice16 : xbsIndex_r4/Slice  nbits=input_bit_width  boolean_output=off  mode=Upper Bit Location + Width  bit1=-0  base1=MSB of Input  bit0=0  base0=MSB of Input  dbl_ovrd=off  block_type=slice
  Slice17 : xbsIndex_r4/Slice  nbits=input_bit_width  boolean_output=off  mode=Upper Bit Location + Width  bit1=-1* input_bit_width  base1=MSB of Input  bit0=0  base0=MSB of Input  dbl_ovrd=off  block_type=slice
  out0 : Outport
  out1 : Outport  Port=2
  wires:
  in/1 -> Slice17/1, Slice16/1
  Reinterpret16/1 -> out1/1
  Slice17/1 -> Reinterpret16/1
  Reinterpret15/1 -> out0/1
  Slice16/1 -> Reinterpret15/1

== system monroe_library/unscr_tail/mirror_spectrum/Subsystem2/cram5 ==
  in0 : Inport
  in1 : Inport  Port=2
  Concat5 : xbsIndex_r4/Concat  num_inputs=2  dbl_ovrd=off  block_type=concat
  Reinterpret23 : xbsIndex_r4/Reinterpret  force_arith_type=on  arith_type=Unsigned  force_bin_pt=on  bin_pt=0  block_type=reinterpret
      settings: infoedit="Changes signal type without altering the binary representation.   You can changed the signal between signed and unsigned, and relocate the binary point.<br><br>Hardware notes: In hardware this block costs nothing.<br><br>Example:  Suppose the input is 6 bits wide, signed, with 2 fractional bits, and the output is forced to unsigned with 0 fractional bits.  Then an input of -2.0 (1110.00 in binary 2's complement) becomes an output of 56 (111000 in binary)."
  Reinterpret24 : xbsIndex_r4/Reinterpret  force_arith_type=on  arith_type=Unsigned  force_bin_pt=on  bin_pt=0  block_type=reinterpret
      settings: infoedit="Changes signal type without altering the binary representation.   You can changed the signal between signed and unsigned, and relocate the binary point.<br><br>Hardware notes: In hardware this block costs nothing.<br><br>Example:  Suppose the input is 6 bits wide, signed, with 2 fractional bits, and the output is forced to unsigned with 0 fractional bits.  Then an input of -2.0 (1110.00 in binary 2's complement) becomes an output of 56 (111000 in binary)."
  out : Outport
  wires:
  Concat5/1 -> out/1
  in0/1 -> Reinterpret23/1
  Reinterpret23/1 -> Concat5/1
  in1/1 -> Reinterpret24/1
  Reinterpret24/1 -> Concat5/2

== system monroe_library/unscr_tail/mirror_spectrum/Subsystem2/uncram6 ==
  in : Inport
  Reinterpret15 : xbsIndex_r4/Reinterpret  force_arith_type=on  arith_type="Signed  (2's comp)"  force_bin_pt=on  bin_pt=input_bit_width-1  block_type=reinterpret
      settings: infoedit="Changes signal type without altering the binary representation.   You can changed the signal between signed and unsigned, and relocate the binary point.<br><br>Hardware notes: In hardware this block costs nothing.<br><br>Example:  Suppose the input is 6 bits wide, signed, with 2 fractional bits, and the output is forced to unsigned with 0 fractional bits.  Then an input of -2.0 (1110.00 in binary 2's complement) becomes an output of 56 (111000 in binary)."
  Reinterpret16 : xbsIndex_r4/Reinterpret  force_arith_type=on  arith_type="Signed  (2's comp)"  force_bin_pt=on  bin_pt=input_bit_width-1  block_type=reinterpret
      settings: infoedit="Changes signal type without altering the binary representation.   You can changed the signal between signed and unsigned, and relocate the binary point.<br><br>Hardware notes: In hardware this block costs nothing.<br><br>Example:  Suppose the input is 6 bits wide, signed, with 2 fractional bits, and the output is forced to unsigned with 0 fractional bits.  Then an input of -2.0 (1110.00 in binary 2's complement) becomes an output of 56 (111000 in binary)."
  Slice16 : xbsIndex_r4/Slice  nbits=input_bit_width  boolean_output=off  mode=Upper Bit Location + Width  bit1=-0  base1=MSB of Input  bit0=0  base0=MSB of Input  dbl_ovrd=off  block_type=slice
  Slice17 : xbsIndex_r4/Slice  nbits=input_bit_width  boolean_output=off  mode=Upper Bit Location + Width  bit1=-1* input_bit_width  base1=MSB of Input  bit0=0  base0=MSB of Input  dbl_ovrd=off  block_type=slice
  out0 : Outport
  out1 : Outport  Port=2
  wires:
  Slice16/1 -> Reinterpret15/1
  Reinterpret15/1 -> out0/1
  Slice17/1 -> Reinterpret16/1
  Reinterpret16/1 -> out1/1
  in/1 -> Slice16/1, Slice17/1

== system monroe_library/unscr_tail/mirror_spectrum/Subsystem3/cram5 ==
  in0 : Inport
  in1 : Inport  Port=2
  Concat5 : xbsIndex_r4/Concat  num_inputs=2  dbl_ovrd=off  block_type=concat
  Reinterpret23 : xbsIndex_r4/Reinterpret  force_arith_type=on  arith_type=Unsigned  force_bin_pt=on  bin_pt=0  block_type=reinterpret
      settings: infoedit="Changes signal type without altering the binary representation.   You can changed the signal between signed and unsigned, and relocate the binary point.<br><br>Hardware notes: In hardware this block costs nothing.<br><br>Example:  Suppose the input is 6 bits wide, signed, with 2 fractional bits, and the output is forced to unsigned with 0 fractional bits.  Then an input of -2.0 (1110.00 in binary 2's complement) becomes an output of 56 (111000 in binary)."
  Reinterpret24 : xbsIndex_r4/Reinterpret  force_arith_type=on  arith_type=Unsigned  force_bin_pt=on  bin_pt=0  block_type=reinterpret
      settings: infoedit="Changes signal type without altering the binary representation.   You can changed the signal between signed and unsigned, and relocate the binary point.<br><br>Hardware notes: In hardware this block costs nothing.<br><br>Example:  Suppose the input is 6 bits wide, signed, with 2 fractional bits, and the output is forced to unsigned with 0 fractional bits.  Then an input of -2.0 (1110.00 in binary 2's complement) becomes an output of 56 (111000 in binary)."
  out : Outport
  wires:
  Reinterpret24/1 -> Concat5/2
  in1/1 -> Reinterpret24/1
  Reinterpret23/1 -> Concat5/1
  in0/1 -> Reinterpret23/1
  Concat5/1 -> out/1
